simulink model "serial_test"  (Simulink 6.4)
settings: Solver=ode4  StartTime=0.0  StopTime=10.0  FixedStep=0.01  RelTol=1e-3
PreLoadFcn:
  | RTWConfigurationCB('preloadfcn', bdroot);
InitFcn:
  | % START RTW CONFIGURATION CODE %
  | RTWConfigurationCB('rtw_target_initfcn',gcs);
  | % END RTW CONFIGURATION CODE %
libraries: mpc555drivers x5, simulink x2
settings Model: LastModifiedBy=Developer  ProdHWDeviceType=Motorola PowerPC
settings OptimizationCC: OptimizeModelRefInitCode=on  LifeSpan=1
settings HardwareCC: ProdIntDivRoundTo=Zero  ProdEndianess=BigEndian  ProdHWDeviceType=Motorola PowerPC
settings RTWCC: SystemTargetFile=mpc555rt.tlc  TemplateMakefile=mpc555rt.tmf  Description=Embedded Target for Motorola MPC555 (real-time target)  ProcessScript=mpc555rt_make_rtw_hook
settings CodeAppCC: IgnoreCustomStorageClasses=off
settings STFCustomTargetCC: TargetFcnLib=codewarrior_tfl_tmw.mat  TargetLibSuffix=.a  TargetPreCompLibLocation=C:\MATLAB\R2006a\toolbox\rtw\targets\mpc555dk\drivers\lib\CODE_WARRIOR  GenFloatMathFcnCalls=ISO_C  CombineOutputUpdateFcns=on  IncludeERTFirstTime=on  ERTCustomFileBanners=on  SupportContinuousTime=off  SupportNonInlinedSFcns=off  SystemTargetFile=mpc555rt.tlc
settings ERTTargetCC: TargetFcnLib=codewarrior_tfl_tmw.mat  TargetPreCompLibLocation=C:\MATLAB\R2006a\toolbox\rtw\targets\mpc555dk\drivers\lib\CODE_WARRIOR  GenFloatMathFcnCalls=ISO_C  IncludeERTFirstTime=on  ERTFirstTimeCompliant=off  InlinedParameterPlacement=NonHierarchical  ERTCustomFileTemplate=example_file_process.tlc  InitialValueSource=Model
settings CustomProperty: DataType=RTWOptions_EnumType__toolbox_rtw_targets_mpc555dk_mpc555dk_mpc555rt_MPC555_OPTIMIZATION_SWITCH  Value=speed
settings EnumStrPairs: String=speed

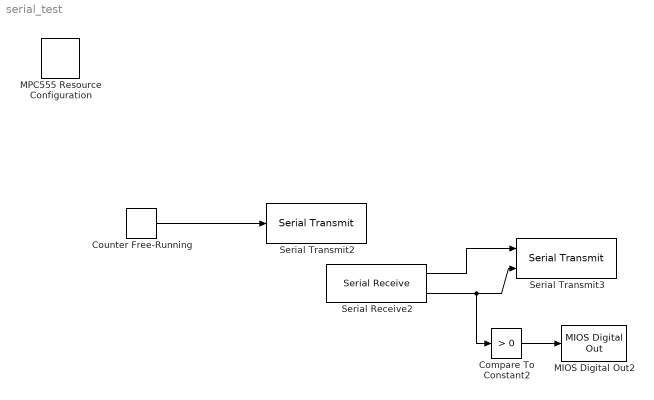
== system serial_test ==
  Compare To Constant2 : simulink/Logic and Bit Operations/Compare To Constant  SystemSampleTime=-1  relop=>  const=0  LogicOutDataTypeMode=boolean  ZeroCross=off
  Counter Free-Running : simulink/Sources/Counter Free-Running  SystemSampleTime=-1  NumBits=8  tsamp=-1
  MIOS Digital Out2 : mpc555drivers/Modular Input//Output System (MIOS1)/MIOS Digital Out  SystemSampleTime=-1  bits=[0]  init=0  t=-1  enablePassThru=off
  MPC555 Resource Configuration : mpc555drivers/MPC555 Resource Configuration  Tag=RTW CONFIGURATION BLOCK  Priority=-100000  SystemSampleTime=-1  oldParentName=serial_test  oldBlockName=|
      | serial_test/MPC555
      | Resource
      | Configuration
  Serial Receive2 : mpc555drivers/Serial Communications Interface (SCI)/Serial Receive  module=1  show_length=off  max_length=1  show_reset=off  show_bytes_read=on  show_flags=off  show_overrun=off  T=0.1
  Serial Transmit2 : mpc555drivers/Serial Communications Interface (SCI)/Serial Transmit  module=1  show_length=off  show_num_sent=off  T=-1
  Serial Transmit3 : mpc555drivers/Serial Communications Interface (SCI)/Serial Transmit  module=2  show_length=on  show_num_sent=off  T=-1
  wires:
  Counter Free-Running/1 -> Serial Transmit2/1
  Compare To Constant2/1 -> MIOS Digital Out2/1
  Serial Receive2/2 -> Compare To Constant2/1, Serial Transmit3/2
  Serial Receive2/1 -> Serial Transmit3/1
